simulink model "CAMFC2_01_WMR01"  (R2017b)
settings: Solver=ode45  StartTime=0.0  StopTime=150  RelTol=1e-3  EnableMultiTasking=on
InitFcn:
  | constant_CAMFC2_01_WMR01
values from neighbouring files (symbols this model uses):
  alpha = 0.1    [constant_CAMFC2_01_WMR01.m]    (also in constant_CAMFC2_04_Comp.m = 0.01; constant_CAMFC2_04_Quad_03.m; constant_CAMFC2_04_Simple.m = 0.01; constant_CAMFC2_04_Simple_DoubleIntegrator.m = 0.01)
  AN = [     0 1 0 0 ... (first row only)    [constant_CAMFC2_01_WMR01.m]    (also in constant_CAMFC2_04_Comp.m = [     0 1 0 0 1; constant_CAMFC2_04_Quad_03.m; constant_CAMFC2_04_Simple.m; constant_CAMFC2_04_Simple_DoubleIntegrator.m)
  B = eye(n)    [constant_CAMFC2_01_WMR01.m]    (also in constant_CAMFC2_04_Quad_03.m; constant_CAMFC2_Quad_New_02.m)
  B_pseudo_inverse = ((B'*B)^(-1))*B'    [constant_CAMFC2_01_WMR01.m]    (also in constant_CAMFC2_Quad_New_02.m)
  BN = [     1 0 0 0 ... (first row only)    [constant_CAMFC2_01_WMR01.m]    (also in constant_CAMFC2_04_Comp.m = [     0 0 0 0 0; constant_CAMFC2_04_Quad_03.m; constant_CAMFC2_04_Simple.m; constant_CAMFC2_04_Simple_DoubleIntegrator.m)
  chi = [0 0 0 0 ... (first row only)    [constant_CAMFC2_01_WMR01.m]    (also in constant_CAMFC2_04_Comp.m = X_m*ones(n0,1); constant_CAMFC2_04_Quad_03.m = X_m*ones(n0,1); constant_CAMFC2_04_Simple.m = X_m*ones(n0,1); constant_CAMFC2_04_Simple_DoubleIntegrator.m = X_m*ones(n0,1))
  Cv = 0.1    [constant_CAMFC2_01_WMR01.m]
  Cw = 0.1    [constant_CAMFC2_01_WMR01.m]
  epsilon_struct = struct('data',epsilon_InitVal)    [constant_CAMFC2_01_WMR01.m]    (also in constant_CAMFC2_04_Comp.m; constant_CAMFC2_04_Quad_03.m; constant_CAMFC2_04_Simple.m; constant_CAMFC2_04_Simple_DoubleIntegrator.m)
  gama1 = 1e4*diag([1e-6*ones(2,1);1e0*ones(2,1)])    [constant_CAMFC2_01_WMR01.m]    (also in constant_CAMFC2_04_Comp.m = 1e+3*diag([1e-6;1e-0]); constant_CAMFC2_04_Quad_03.m = 1e+2*diag(1e-0*ones(n0,1)); constant_CAMFC2_04_Simple.m = 1e+2*diag([1e-0;1e-0]); constant_CAMFC2_04_Simple_Formation.m = 1e+2*diag([1e-0;1e-0]))
  gama2 = 1e-2*diag([1e-6*ones(2,1);1e0*ones(2,1)])    [constant_CAMFC2_01_WMR01.m]    (also in constant_CAMFC2_04_Comp.m = 1e+0*diag([1e-6;1e-0]); constant_CAMFC2_04_Quad_03.m = 1e+0*diag(1e-0*ones(n0,1)); constant_CAMFC2_04_Simple.m = 1e+1*diag([1e-0;1e-0]); constant_CAMFC2_04_Simple_Formation.m = 1e+1*diag([1e-0;1e-0]))
  H = L + BN    [constant_CAMFC2_01_WMR01.m]    (also in constant_CAMFC2_04_Comp.m; constant_CAMFC2_04_Quad_03.m; constant_CAMFC2_04_Simple.m; constant_CAMFC2_04_Simple_DoubleIntegrator.m)
  J = 0.01    [constant_CAMFC2_01_WMR01.m]    (also in constant_CAMFC2_04_Quad_03.m = 1.0e-3 * diag([1 1 2],0); constant_CAMFC2_Quad_New_02.m = 1.2416e-3 * diag([1 1 2],0))
  K = 1e-2*eye(n)    [constant_CAMFC2_01_WMR01.m]    (also in constant_CAMFC2_Quad_New_02.m = 1e+1*eye(n))
  k1 = 1    [constant_CAMFC2_01_WMR01.m]    (also in constant_CAMFC2_04_Comp.m; constant_CAMFC2_04_Quad_03.m = 50; constant_CAMFC2_04_Simple.m; constant_CAMFC2_04_Simple_DoubleIntegrator.m)
  k2 = 1    [constant_CAMFC2_01_WMR01.m]    (also in constant_CAMFC2_04_Comp.m; constant_CAMFC2_04_Quad_03.m; constant_CAMFC2_04_Simple.m; constant_CAMFC2_04_Simple_DoubleIntegrator.m)
  L0 = 0.1    [constant_CAMFC2_01_WMR01.m]
  M = 1    [constant_CAMFC2_01_WMR01.m]    (also in constant_CAMFC2_04_Quad_03.m = 2; constant_CAMFC2_Quad_New_02.m = 2)
  N = 4    [constant_CAMFC2_01_WMR01.m]    (also in constant_CAMFC2_04_Comp.m = 5; constant_CAMFC2_04_Quad_03.m; constant_CAMFC2_04_Simple.m; constant_CAMFC2_04_Simple_DoubleIntegrator.m)
  n = 4    [constant_CAMFC2_01_WMR01.m]    (also in constant_CAMFC2_04_Comp.m = 2; constant_CAMFC2_04_Quad_03.m = 6; constant_CAMFC2_04_Simple.m = 2; constant_CAMFC2_04_Simple_DoubleIntegrator.m = 2)
  n0 = 2    [constant_CAMFC2_01_WMR01.m]    (also in constant_CAMFC2_04_Comp.m = 1; constant_CAMFC2_04_Quad_03.m = 3; constant_CAMFC2_04_Simple.m; constant_CAMFC2_04_Simple_DoubleIntegrator.m = 1)
  Observer_Gain = 100    [constant_CAMFC2_01_WMR01.m]    (also in constant_CAMFC2_04_Comp.m = 10; constant_CAMFC2_04_Quad_03.m = 1; constant_CAMFC2_04_Simple.m; constant_CAMFC2_04_Simple_DoubleIntegrator.m)
  Observer_Gain1 = 100    [constant_CAMFC2_01_WMR01.m]    (also in constant_CAMFC2_04_Comp.m = 10; constant_CAMFC2_04_Quad_03.m = 1; constant_CAMFC2_04_Simple.m; constant_CAMFC2_04_Simple_DoubleIntegrator.m)
  P_struct = struct('data',P_InitVal)    [constant_CAMFC2_01_WMR01.m]    (also in constant_CAMFC2_04_Comp.m; constant_CAMFC2_04_Quad_03.m; constant_CAMFC2_04_Simple.m; constant_CAMFC2_04_Simple_DoubleIntegrator.m)
  Q = 1e-0*eye(n)    [constant_CAMFC2_01_WMR01.m]    (also in constant_CAMFC2_04_Comp.m = 1.0e+2*eye(n); constant_CAMFC2_04_Quad_03.m = 1e-0*eye(n0); constant_CAMFC2_04_Simple.m = 1.0e+1*eye(n); constant_CAMFC2_04_Simple_Formation.m = 1.0e+1*eye(n))
  R = 1e-0*eye(n)    [constant_CAMFC2_01_WMR01.m]    (also in constant_CAMFC2_04_Quad_03.m; constant_CAMFC2_Quad_New_02.m = 1e+0*eye(n))
  R0 = 0.1    [constant_CAMFC2_01_WMR01.m]
  rho1 = 1e-1    (= 0.1)    [constant_CAMFC2_01_WMR01.m]    (also in constant_CAMFC2_04_Comp.m = 1; constant_CAMFC2_04_Quad_03.m = 1; constant_CAMFC2_04_Simple.m = 1; constant_CAMFC2_04_Simple_DoubleIntegrator.m = 1)
  rho2 = 1e-3    (= 0.001)    [constant_CAMFC2_01_WMR01.m]    (also in constant_CAMFC2_04_Comp.m = 1; constant_CAMFC2_04_Quad_03.m = 1; constant_CAMFC2_04_Simple.m = 1; constant_CAMFC2_04_Simple_DoubleIntegrator.m = 10)
  T_struct = struct('data',T_InitVal)    [constant_CAMFC2_01_WMR01.m]    (also in constant_CAMFC2_04_Comp.m; constant_CAMFC2_04_Quad_03.m; constant_CAMFC2_04_Simple.m; constant_CAMFC2_04_Simple_DoubleIntegrator.m)
  Thresh = 1e-4    (= 0.0001)    [constant_CAMFC2_01_WMR01.m]
  U_dot0_M = U_dot0_m*ones(n,1)    [constant_CAMFC2_01_WMR01.m]    (also in constant_CAMFC2_Quad_New_02.m = U_dot0_m*ones(n0,1))
  Upsilon_M = Upsilon_m*ones(n,1)    [constant_CAMFC2_01_WMR01.m]    (also in constant_CAMFC2_04_Comp.m; constant_CAMFC2_04_Quad_03.m = Upsilon_m*ones(n0,1); constant_CAMFC2_04_Simple.m; constant_CAMFC2_04_Simple_DoubleIntegrator.m)
libraries: simulink x1
(part 2 of 2)

== matlab function CAMFC2_01_WMR01/Agent #1/Decenteralized Cooperaive Controller #1/Differentiator2/Sliding differentiator ==
  data: u output; u1 input; e input; k1 parameter; alpha parameter
function u = fcn(u1,e,k1,alpha)

b=k1;

ABS = abs(e);
SGN = e ./ (ABS + alpha);
u = u1 - b*((ABS.^0.5).*SGN); 

end

== matlab function CAMFC2_01_WMR01/Agent #1/Decenteralized Cooperaive Controller #1/Differentiator2/Sliding differentiator1 ==
  data: Du1 output; e input; k2 parameter; alpha parameter
function Du1 = fcn(e,k2,alpha)

a=k2;

ABS = abs(e);
SGN = e ./ (ABS + alpha);
Du1 = - a*SGN;

end

== matlab function CAMFC2_01_WMR01/Agent #1/WMR Plant-01/WMR model ==
  data: X input; u1 input; DX output; u2 input; t input; Cv parameter; Cw parameter; M parameter; J parameter; R0 parameter; L0 parameter
function DX = fcn(X,u1,u2,t,Cv,Cw,M,J,R0,L0)

x = X(1);
y = X(2);
T = X(3);
v = X(4);
w = X(5);

T1 = 0.01 * u1; 
T2 = 0.01 * u2; 

F = (1/R0)*(T1+T2);
Tau = (L0/R0)*(T1-T2);

Dv = (F - Cv*v + (0*sin(1*t)))/M ;
Dw = (Tau - Cw*w + (0*sin(1*t)))/J ;

Dx = v*cos(T);
Dy = v*sin(T);
DT = w;

DX = [Dx Dy DT Dv Dw]';

end

== matlab function CAMFC2_01_WMR01/Agent #2/Controller interpreter ==
  data: u output; U input
function u = fcn(U)

U1 = U(3);
U2 = U(4); 

u1 = 0.5 * (U1+U2);
u2 = 0.5 * (U1-U2);

u = [u1;u2];

end

== matlab function CAMFC2_01_WMR01/Agent #1/Decenteralized Cooperaive Controller #1/Main Controller #1 ==
  data: n parameter; n0 parameter; U output; R parameter; Q parameter; P_i input; e_i input; K parameter; Zeta_i input; BN parameter; A_hat_i input; u0 input; z0 input; DT_i input; T_i input; N parameter; H parameter; B parameter; g_hat input; Approx_U input; Agent_Num input; B_pseudo_inverse parameter; ui input; x input
function U = fcn(n,n0,R,Q,P_i,e_i,K,Zeta_i,BN,A_hat_i,u0,z0,DT_i,T_i,N,H,B,g_hat,Approx_U,Agent_Num,B_pseudo_inverse,ui,x)

D_eta_0 = DT_i(1,:)';

%%
z0_i = [z0;ui(1:n0)];
u0_i = u0;

%%
U2 = 1/2 * R * P_i * e_i; %Consensus Error
U6 = - BN(Agent_Num,Agent_Num)*(D_eta_0 - u0_i); %Connection to the leader
U7 = K * Zeta_i; %Consensus time-integral

U1 = zeros(n,1);
U3 = BN(Agent_Num,Agent_Num)*z0_i - e_i;
U4 = zeros(n,1);
U5 = zeros(n,1);
for i=1:N      
    if i~= Agent_Num
        U1 = U1 - (H(Agent_Num,i)*B*Approx_U((i-1)*n+1:(i*n),1)); %Observer on leader
    end
    U3 = U3 + (H(Agent_Num,i)*(2*x((i-1)*n+1:(i*n),1)) - T_i(i+1,:)'); %Formation parameters  
    U4 = U4 - (H(Agent_Num,i)*g_hat((i-1)*n+1:(i*n),1)); %nonlinear compensation 
    U5 = U5 + (H(Agent_Num,i)*DT_i(i+1,:)'); %Derivative of Formation parameters  
end
U3 = -A_hat_i * U3;
U8 = (2*Q - 3/4*R*P_i)*e_i;

U_input = U1 + U2 + U3 + U4 + U5 + U6 + U7 + U8;

U = B_pseudo_inverse * U_input / H(Agent_Num,Agent_Num);

end

== matlab function CAMFC2_01_WMR01/Agent #1/Decenteralized Cooperaive Controller #1/Module to compute Consensus Error #1 ==
  data: T_i input; xi input; x input; x0 input; ep output; AN parameter; BN parameter; N parameter; n parameter; n0 parameter; Agent_Num input; ui input; u0 input; Thresh parameter; xmi output; xm0 output; Td_in input; Td output
function [ep,xmi,xm0,Td] = fcn(T_i,xi,x,x0,AN,BN,N,n,n0,Agent_Num,ui,u0,Thresh,Td_in)

Diff_Star_to0 = (T_i((Agent_Num+1),:))';
Diff_Star_to_Other = (eye(n) * Diff_Star_to0 * ones(1,N))' - T_i(2:N+1,:);
Diff_Star_to_Other = Diff_Star_to_Other';

xp = zeros(n+1,N);
for i=1:N
    xp(1:n+1,i) = x((i-1)*(n+1)+1:(i*(n+1)));
end

%% variables modification

Ta = xi(3);
Td0 = Td_in(1);
if (abs(u0(1))+abs(u0(2))) > (1*Thresh)
    y_Err = (x0(2)-xi(2));
    x_Err = (x0(1)-xi(1));
    XS = (y_Err/x_Err);
    Td0 = atan(XS); 
    if abs(Td0)>1.5
        Td0 = abs(Td0);
    end
end

%Td = zeros(N+1,1);
%Td(1) = Td0;
Td = Td0;
Diff_Real = zeros(n,N);
Dxi = zeros(2,N);
for i=1:N
    Diff_Real(1,i) = (xp(1,Agent_Num) - xp(1,i))*cos(Ta) + (xp(2,Agent_Num) - xp(2,i))*sin(Ta);
%    Tdi = Td_in(i+1);
%     Dxi(1,i) = xp(4,i)*cos(xp(3,i));
%     Dxi(2,i) = xp(4,i)*sin(xp(3,i));
%     if (abs(Dxi(1,i))+abs(Dxi(2,i))) > Thresh
%         y_Erri = xp(2,Agent_Num) - xp(2,i);
%         x_Erri = xp(1,Agent_Num) - xp(1,i);
%         Tdi = atan(y_Erri/x_Erri);
%         if abs(Tdi)>1.5
%             Tdi = abs(Tdi);
%         end
%     end
%    Diff_Real(2,i) = Ta - Tdi;
    Diff_Real(2,i) = Ta - xp(3,i);
    Diff_Real(3:4,i) = xp(4:5,Agent_Num) - xp(4:5,i); 
%    Td(i+1) = Tdi;
end
Diff_Real0 = zeros(n,1);
Diff_Real0(1) = (xp(1,Agent_Num) - x0(1))*cos(Ta) + (xp(2,Agent_Num) - x0(2))*sin(Ta);
Diff_Real0(2) = Ta - Td0; 
Diff_Real0(3:4) = xp(4:5,Agent_Num) - ui(1:n0);

Posi = xi(1)*cos(Ta) + xi(2)*sin(Ta);
Posd = x0(1)*cos(Ta) + x0(2)*sin(Ta);
xmi = [Posi;Ta;xi(4);xi(5)];
xm0 = [Posd;Td0]; 

%%

ep = zeros(n,1);
ep(1:2,1) = ep(1:2,1) + ( BN(Agent_Num,Agent_Num)*(-Diff_Real0(1:2)+Diff_Star_to0(1:2)) );
ep(3:4,1) = ep(3:4,1) + ( 1*(-Diff_Real0(3:4)+Diff_Star_to0(3:4)) );
for i=1:N            
    ep(1:n,1) = ep(1:n,1) + AN(Agent_Num,i)*(-Diff_Real(:,i)+Diff_Star_to_Other(:,i));
end

end

== matlab function CAMFC2_01_WMR01/Agent #1/Decenteralized Cooperaive Controller #1/Observer T#1 ==
  data: T_struct parameter; T input; DT_i output; epsilon input; epsilon_struct parameter; H parameter; BN parameter; AN parameter; T_i input; chi parameter; Upsilon_M parameter; epsilon_i output; N parameter; n parameter; Agent_Num input; Observer_Gain1 parameter
function [DT_i,epsilon_i] = fcn(T_struct,T,epsilon,epsilon_struct,H,BN,AN,T_i,chi,Upsilon_M,N,n,Agent_Num,Observer_Gain1)

T_struct(1).data = T.t1;
T_struct(2).data = T.t2;
T_struct(3).data = T.t3;
T_struct(4).data = T.t4;

epsilon_struct(1).data = epsilon.eps1;
epsilon_struct(2).data = epsilon.eps2;
epsilon_struct(3).data = epsilon.eps3;
epsilon_struct(4).data = epsilon.eps4;

epsilon_i = + BN(Agent_Num,Agent_Num)*(T_i - chi);
Sum2 = zeros(N+1,n);
for i=1:N
    epsilon_i = epsilon_i + ( AN(Agent_Num,i) * (T_i - T_struct(i).data) );  
    Sum2 = Sum2 + ( H(i,Agent_Num) * epsilon_struct(i).data );
end

Sum21 = abs(Sum2) + 0.1;
SGN2 = Sum2./Sum21;

DT_i = -Observer_Gain1*epsilon_i - SGN2*diag(Upsilon_M);

end

== matlab function CAMFC2_01_WMR01/Agent #1/Decenteralized Cooperaive Controller #1/Observer q#1 ==
  data: q input; Dq_i output; tau input; H parameter; BN parameter; AN parameter; q_i input; u0 input; U_dot0_M parameter; tau_i output; N parameter; Agent_Num input; Observer_Gain parameter; n parameter
function [Dq_i,tau_i] = fcn(q,tau,H,BN,AN,q_i,u0,U_dot0_M,N,Agent_Num,Observer_Gain,n)

tau_i = + BN(Agent_Num,Agent_Num)*(q_i - u0);
Sum2 = zeros(n,1);
for i=1:N
    tau_i = tau_i + ( AN(Agent_Num,i) * (q_i - q(((i-1)*n+1):n*i)) );  
    Sum2 = Sum2 + ( H(i,Agent_Num) * tau(((i-1)*n+1):n*i) );
end

Sum21 = abs(Sum2) + 0.01;
SGN2 = Sum2./Sum21;

Dq_i = -Observer_Gain*tau_i - diag(SGN2)*U_dot0_M;

end

== matlab function CAMFC2_01_WMR01/Agent #1/Decenteralized Cooperaive Controller #1/DRE ==
  data: P input; A_hat input; B parameter; R parameter; DP output; Q parameter
function DP = fcn(P,A_hat,B,R,Q)

DP = 2*A_hat*P + 2*P*A_hat' - P*B*R*B'*P + 2*Q;

end

== matlab function CAMFC2_01_WMR01/Agent #2/WMR Plant-02/WMR model ==
  data: X input; u1 input; DX output; u2 input; t input; Cv parameter; Cw parameter; M parameter; J parameter; R0 parameter; L0 parameter
function DX = fcn(X,u1,u2,t,Cv,Cw,M,J,R0,L0)

x = X(1);
y = X(2);
T = X(3);
v = X(4);
w = X(5);

T1 = 0.01 * u1; 
T2 = 0.01 * u2; 

F = (1/R0)*(T1+T2);
Tau = (L0/R0)*(T1-T2);

Dv = (F - Cv*v + (0*sin(1*t)))/M ;
Dw = (Tau - Cw*w + (0*sin(1*t)))/J ;

Dx = v*cos(T);
Dy = v*sin(T);
DT = w;

DX = [Dx Dy DT Dv Dw]';

end

== matlab function CAMFC2_01_WMR01/Agent #3/Controller interpreter ==
  data: u output; U input
function u = fcn(U)

U1 = U(3);
U2 = U(4); 

u1 = 0.5 * (U1+U2);
u2 = 0.5 * (U1-U2);

u = [u1;u2];

end

== matlab function CAMFC2_01_WMR01/Agent #2/Decenteralized Cooperaive Controller #2/Adaptive Law A#2 ==
  data: Agent_Num input; A_hat input; gama2 parameter; rho2 parameter; T_i input; P_i input; DA_hat output; e_i input; H parameter; BN parameter; N parameter; n parameter; n0 parameter; z0 input; x input; ui input
function DA_hat = fcn(Agent_Num,A_hat,gama2,rho2,T_i,P_i,e_i,H,BN,N,n,n0,z0,x,ui)

%% 
z0_i = [z0;ui(1:n0)]; 

%%
vA_hat = diag(A_hat);

Sum = zeros(n,1);
for i=2:(N+1)
    Sum = Sum + (H(Agent_Num,(i-1)) * (2*x(((i-1)-1)*n+1:((i-1)*n),1)) - T_i(i,:)');
end
Sum = Sum + BN(Agent_Num,Agent_Num)*z0_i - e_i;
    
DvA_hat = -gama2*diag(Sum)*P_i * e_i - (rho2*gama2*vA_hat);

DA_hat = diag(DvA_hat);

end

== matlab function CAMFC2_01_WMR01/Agent #2/Decenteralized Cooperaive Controller #2/Adaptive Law g#2 ==
  data: Agent_Num input; g_hat input; gama1 parameter; rho1 parameter; P input; P_struct parameter; Dg_hat output; e input; H parameter; N parameter; n parameter
function Dg_hat = fcn(Agent_Num,g_hat,gama1,rho1,P,P_struct,e,H,N,n)

P_struct(1).data = P.p1;
P_struct(2).data = P.p2;
P_struct(3).data = P.p3;
P_struct(4).data = P.p4;

Sum = zeros(n,1);
for i=1:N  
    Sum = Sum + (H(i,Agent_Num) * P_struct(i).data * e((i-1)*n+1:(i*n),1)); %Adaptive law
end
    
Dg_hat = -gama1*Sum - (rho1*gama1*g_hat);

end

== matlab function CAMFC2_01_WMR01/Agent #2/Decenteralized Cooperaive Controller #2/Approx. U#2 ==
  data: Agent_Num input; q_i input; DT_i input; Approx_U_i output; B_pseudo_inverse parameter; A_hat_i input; x_i input; g_hat_i input
function Approx_U_i  = fcn(Agent_Num,q_i,DT_i,B_pseudo_inverse,A_hat_i,x_i,g_hat_i)

D_eta_0 = DT_i(1,:)';
D_eta_i = DT_i(Agent_Num,:)';

u0_i = q_i;

Approx_U_i = B_pseudo_inverse * (u0_i - A_hat_i * x_i - g_hat_i + D_eta_i - D_eta_0);

end

== matlab function CAMFC2_01_WMR01/Agent #2/Decenteralized Cooperaive Controller #2/DRE ==
  data: P input; A_hat input; B parameter; R parameter; DP output; Q parameter
function DP = fcn(P,A_hat,B,R,Q)

DP = 2*A_hat*P + 2*P*A_hat' - P*B*R*B'*P + 2*Q;

end

== matlab function CAMFC2_01_WMR01/Agent #1/Decenteralized Cooperaive Controller #1/Differentiator1/Sliding differentiator ==
  data: u output; u1 input; e input; k1 parameter; alpha parameter
function u = fcn(u1,e,k1,alpha)

b=k1;

ABS = abs(e);
SGN = e ./ (ABS + alpha);
u = u1 - b*((ABS.^0.5).*SGN); 

end

== matlab function CAMFC2_01_WMR01/Agent #1/Decenteralized Cooperaive Controller #1/Differentiator1/Sliding differentiator1 ==
  data: Du1 output; e input; k2 parameter; alpha parameter
function Du1 = fcn(e,k2,alpha)

a=k2;

ABS = abs(e);
SGN = e ./ (ABS + alpha);
Du1 = - a*SGN;

end

== matlab function CAMFC2_01_WMR01/Agent #3/WMR Plant-03/WMR model ==
  data: X input; u1 input; DX output; u2 input; t input; Cv parameter; Cw parameter; M parameter; J parameter; R0 parameter; L0 parameter
function DX = fcn(X,u1,u2,t,Cv,Cw,M,J,R0,L0)

x = X(1);
y = X(2);
T = X(3);
v = X(4);
w = X(5);

T1 = 0.01 * u1; 
T2 = 0.01 * u2; 

F = (1/R0)*(T1+T2);
Tau = (L0/R0)*(T1-T2);

Dv = (F - Cv*v + (0*sin(1*t)))/M ;
Dw = (Tau - Cw*w + (0*sin(1*t)))/J ;

Dx = v*cos(T);
Dy = v*sin(T);
DT = w;

DX = [Dx Dy DT Dv Dw]';

end

== matlab function CAMFC2_01_WMR01/Agent #4/Controller interpreter ==
  data: u output; U input
function u = fcn(U)

U1 = U(3);
U2 = U(4); 

u1 = 0.5 * (U1+U2);
u2 = 0.5 * (U1-U2);

u = [u1;u2];

end

== matlab function CAMFC2_01_WMR01/Agent #2/Decenteralized Cooperaive Controller #2/Differentiator0/Sliding differentiator ==
  data: u output; u1 input; e input; k1 parameter; alpha parameter
function u = fcn(u1,e,k1,alpha)

b=k1;

ABS = abs(e);
SGN = e ./ (ABS + alpha);
u = u1 - b*((ABS.^0.5).*SGN); 

end

== matlab function CAMFC2_01_WMR01/Agent #2/Decenteralized Cooperaive Controller #2/Differentiator0/Sliding differentiator1 ==
  data: Du1 output; e input; k2 parameter; alpha parameter
function Du1 = fcn(e,k2,alpha)

a=k2;

ABS = abs(e);
SGN = e ./ (ABS + alpha);
Du1 = - a*SGN;

end

== matlab function CAMFC2_01_WMR01/Agent #2/Decenteralized Cooperaive Controller #2/Differentiator1/Sliding differentiator ==
  data: u output; u1 input; e input; k1 parameter; alpha parameter
function u = fcn(u1,e,k1,alpha)

b=k1;

ABS = abs(e);
SGN = e ./ (ABS + alpha);
u = u1 - b*((ABS.^0.5).*SGN); 

end

== matlab function CAMFC2_01_WMR01/Agent #2/Decenteralized Cooperaive Controller #2/Differentiator1/Sliding differentiator1 ==
  data: Du1 output; e input; k2 parameter; alpha parameter
function Du1 = fcn(e,k2,alpha)

a=k2;

ABS = abs(e);
SGN = e ./ (ABS + alpha);
Du1 = - a*SGN;

end

== matlab function CAMFC2_01_WMR01/Agent #4/WMR Plant-04/WMR model ==
  data: X input; u1 input; DX output; u2 input; t input; Cv parameter; Cw parameter; M parameter; J parameter; R0 parameter; L0 parameter
function DX = fcn(X,u1,u2,t,Cv,Cw,M,J,R0,L0)

x = X(1);
y = X(2);
T = X(3);
v = X(4);
w = X(5);

T1 = 0.01 * u1; 
T2 = 0.01 * u2; 

F = (1/R0)*(T1+T2);
Tau = (L0/R0)*(T1-T2);

Dv = (F - Cv*v + (0*sin(1*t)))/M ;
Dw = (Tau - Cw*w + (0*sin(1*t)))/J ;

Dx = v*cos(T);
Dy = v*sin(T);
DT = w;

DX = [Dx Dy DT Dv Dw]';

end

== matlab function CAMFC2_01_WMR01/Agent #2/Decenteralized Cooperaive Controller #2/Differentiator2/Sliding differentiator ==
  data: u output; u1 input; e input; k1 parameter; alpha parameter
function u = fcn(u1,e,k1,alpha)

b=k1;

ABS = abs(e);
SGN = e ./ (ABS + alpha);
u = u1 - b*((ABS.^0.5).*SGN); 

end

== matlab function CAMFC2_01_WMR01/Agent #3/Decenteralized Cooperaive Controller #3/Adaptive Law A#3 ==
  data: Agent_Num input; A_hat input; gama2 parameter; rho2 parameter; T_i input; P_i input; DA_hat output; e_i input; H parameter; BN parameter; N parameter; n parameter; n0 parameter; z0 input; x input; ui input
function DA_hat = fcn(Agent_Num,A_hat,gama2,rho2,T_i,P_i,e_i,H,BN,N,n,n0,z0,x,ui)

%% 
z0_i = [z0;ui(1:n0)]; 

%%
vA_hat = diag(A_hat);

Sum = zeros(n,1);
for i=2:(N+1)
    Sum = Sum + (H(Agent_Num,(i-1)) * (2*x(((i-1)-1)*n+1:((i-1)*n),1)) - T_i(i,:)');
end
Sum = Sum + BN(Agent_Num,Agent_Num)*z0_i - e_i;
    
DvA_hat = -gama2*diag(Sum)*P_i * e_i - (rho2*gama2*vA_hat);

DA_hat = diag(DvA_hat);

end

== matlab function CAMFC2_01_WMR01/Agent #3/Decenteralized Cooperaive Controller #3/Adaptive Law g#3 ==
  data: Agent_Num input; g_hat input; gama1 parameter; rho1 parameter; P input; P_struct parameter; Dg_hat output; e input; H parameter; N parameter; n parameter
function Dg_hat = fcn(Agent_Num,g_hat,gama1,rho1,P,P_struct,e,H,N,n)

P_struct(1).data = P.p1;
P_struct(2).data = P.p2;
P_struct(3).data = P.p3;
P_struct(4).data = P.p4;

Sum = zeros(n,1);
for i=1:N  
    Sum = Sum + (H(i,Agent_Num) * P_struct(i).data * e((i-1)*n+1:(i*n),1)); %Adaptive law
end
    
Dg_hat = -gama1*Sum - (rho1*gama1*g_hat);

end

== matlab function CAMFC2_01_WMR01/Agent #3/Decenteralized Cooperaive Controller #3/Approx. U#3 ==
  data: Agent_Num input; q_i input; DT_i input; Approx_U_i output; B_pseudo_inverse parameter; A_hat_i input; x_i input; g_hat_i input
function Approx_U_i  = fcn(Agent_Num,q_i,DT_i,B_pseudo_inverse,A_hat_i,x_i,g_hat_i)

D_eta_0 = DT_i(1,:)';
D_eta_i = DT_i(Agent_Num,:)';

u0_i = q_i;

Approx_U_i = B_pseudo_inverse * (u0_i - A_hat_i * x_i - g_hat_i + D_eta_i - D_eta_0);

end

== matlab function CAMFC2_01_WMR01/Agent #3/Decenteralized Cooperaive Controller #3/DRE ==
  data: P input; A_hat input; B parameter; R parameter; DP output; Q parameter
function DP = fcn(P,A_hat,B,R,Q)

DP = 2*A_hat*P + 2*P*A_hat' - P*B*R*B'*P + 2*Q;

end

== matlab function CAMFC2_01_WMR01/Agent #2/Decenteralized Cooperaive Controller #2/Differentiator2/Sliding differentiator1 ==
  data: Du1 output; e input; k2 parameter; alpha parameter
function Du1 = fcn(e,k2,alpha)

a=k2;

ABS = abs(e);
SGN = e ./ (ABS + alpha);
Du1 = - a*SGN;

end

== matlab function CAMFC2_01_WMR01/Agent #2/Decenteralized Cooperaive Controller #2/Main Controller #2 ==
  data: n parameter; n0 parameter; U output; R parameter; Q parameter; P_i input; e_i input; K parameter; Zeta_i input; BN parameter; A_hat_i input; u0 input; z0 input; DT_i input; T_i input; N parameter; H parameter; B parameter; g_hat input; Approx_U input; Agent_Num input; B_pseudo_inverse parameter; ui input; x input
function U = fcn(n,n0,R,Q,P_i,e_i,K,Zeta_i,BN,A_hat_i,u0,z0,DT_i,T_i,N,H,B,g_hat,Approx_U,Agent_Num,B_pseudo_inverse,ui,x)

D_eta_0 = DT_i(1,:)';

%%
z0_i = [z0;ui(1:n0)];
u0_i = u0;

%%
U2 = 1/2 * R * P_i * e_i; %Consensus Error
U6 = - BN(Agent_Num,Agent_Num)*(D_eta_0 - u0_i); %Connection to the leader
U7 = K * Zeta_i; %Consensus time-integral

U1 = zeros(n,1);
U3 = BN(Agent_Num,Agent_Num)*z0_i - e_i;
U4 = zeros(n,1);
U5 = zeros(n,1);
for i=1:N      
    if i~= Agent_Num
        U1 = U1 - (H(Agent_Num,i)*B*Approx_U((i-1)*n+1:(i*n),1)); %Observer on leader
    end
    U3 = U3 + (H(Agent_Num,i)*(2*x((i-1)*n+1:(i*n),1)) - T_i(i+1,:)'); %Formation parameters  
    U4 = U4 - (H(Agent_Num,i)*g_hat((i-1)*n+1:(i*n),1)); %nonlinear compensation 
    U5 = U5 + (H(Agent_Num,i)*DT_i(i+1,:)'); %Derivative of Formation parameters  
end
U3 = -A_hat_i * U3;
U8 = (2*Q - 3/4*R*P_i)*e_i;

U_input = U1 + U2 + U3 + U4 + U5 + U6 + U7 + U8;

U = B_pseudo_inverse * U_input / H(Agent_Num,Agent_Num);

end

== matlab function CAMFC2_01_WMR01/Agent #1/Decenteralized Cooperaive Controller #1/Differentiator0/Sliding differentiator ==
  data: u output; u1 input; e input; k1 parameter; alpha parameter
function u = fcn(u1,e,k1,alpha)

b=k1;

ABS = abs(e);
SGN = e ./ (ABS + alpha);
u = u1 - b*((ABS.^0.5).*SGN); 

end

== matlab function CAMFC2_01_WMR01/Agent #1/Decenteralized Cooperaive Controller #1/Differentiator0/Sliding differentiator1 ==
  data: Du1 output; e input; k2 parameter; alpha parameter
function Du1 = fcn(e,k2,alpha)

a=k2;

ABS = abs(e);
SGN = e ./ (ABS + alpha);
Du1 = - a*SGN;

end

== matlab function CAMFC2_01_WMR01/Agent #3/Decenteralized Cooperaive Controller #3/Differentiator0/Sliding differentiator ==
  data: u output; u1 input; e input; k1 parameter; alpha parameter
function u = fcn(u1,e,k1,alpha)

b=k1;

ABS = abs(e);
SGN = e ./ (ABS + alpha);
u = u1 - b*((ABS.^0.5).*SGN); 

end

== matlab function CAMFC2_01_WMR01/Agent #3/Decenteralized Cooperaive Controller #3/Differentiator0/Sliding differentiator1 ==
  data: Du1 output; e input; k2 parameter; alpha parameter
function Du1 = fcn(e,k2,alpha)

a=k2;

ABS = abs(e);
SGN = e ./ (ABS + alpha);
Du1 = - a*SGN;

end

== matlab function CAMFC2_01_WMR01/Agent #3/Decenteralized Cooperaive Controller #3/Differentiator1/Sliding differentiator ==
  data: u output; u1 input; e input; k1 parameter; alpha parameter
function u = fcn(u1,e,k1,alpha)

b=k1;

ABS = abs(e);
SGN = e ./ (ABS + alpha);
u = u1 - b*((ABS.^0.5).*SGN); 

end

== matlab function CAMFC2_01_WMR01/Agent #3/Decenteralized Cooperaive Controller #3/Differentiator1/Sliding differentiator1 ==
  data: Du1 output; e input; k2 parameter; alpha parameter
function Du1 = fcn(e,k2,alpha)

a=k2;

ABS = abs(e);
SGN = e ./ (ABS + alpha);
Du1 = - a*SGN;

end

== matlab function CAMFC2_01_WMR01/Agent #3/Decenteralized Cooperaive Controller #3/Differentiator2/Sliding differentiator ==
  data: u output; u1 input; e input; k1 parameter; alpha parameter
function u = fcn(u1,e,k1,alpha)

b=k1;

ABS = abs(e);
SGN = e ./ (ABS + alpha);
u = u1 - b*((ABS.^0.5).*SGN); 

end

== matlab function CAMFC2_01_WMR01/Agent #3/Decenteralized Cooperaive Controller #3/Differentiator2/Sliding differentiator1 ==
  data: Du1 output; e input; k2 parameter; alpha parameter
function Du1 = fcn(e,k2,alpha)

a=k2;

ABS = abs(e);
SGN = e ./ (ABS + alpha);
Du1 = - a*SGN;

end

== matlab function CAMFC2_01_WMR01/Agent #4/Decenteralized Cooperaive Controller #4/Adaptive Law A#4 ==
  data: Agent_Num input; A_hat input; gama2 parameter; rho2 parameter; T_i input; P_i input; DA_hat output; e_i input; H parameter; BN parameter; N parameter; n parameter; n0 parameter; z0 input; x input; ui input
function DA_hat = fcn(Agent_Num,A_hat,gama2,rho2,T_i,P_i,e_i,H,BN,N,n,n0,z0,x,ui)

%% 
z0_i = [z0;ui(1:n0)]; 

%%
vA_hat = diag(A_hat);

Sum = zeros(n,1);
for i=2:(N+1)
    Sum = Sum + (H(Agent_Num,(i-1)) * (2*x(((i-1)-1)*n+1:((i-1)*n),1)) - T_i(i,:)');
end
Sum = Sum + BN(Agent_Num,Agent_Num)*z0_i - e_i;
    
DvA_hat = -gama2*diag(Sum)*P_i * e_i - (rho2*gama2*vA_hat);

DA_hat = diag(DvA_hat);

end

== matlab function CAMFC2_01_WMR01/Agent #4/Decenteralized Cooperaive Controller #4/Adaptive Law g#4 ==
  data: Agent_Num input; g_hat input; gama1 parameter; rho1 parameter; P input; P_struct parameter; Dg_hat output; e input; H parameter; N parameter; n parameter
function Dg_hat = fcn(Agent_Num,g_hat,gama1,rho1,P,P_struct,e,H,N,n)

P_struct(1).data = P.p1;
P_struct(2).data = P.p2;
P_struct(3).data = P.p3;
P_struct(4).data = P.p4;

Sum = zeros(n,1);
for i=1:N  
    Sum = Sum + (H(i,Agent_Num) * P_struct(i).data * e((i-1)*n+1:(i*n),1)); %Adaptive law
end
    
Dg_hat = -gama1*Sum - (rho1*gama1*g_hat);

end

== matlab function CAMFC2_01_WMR01/Agent #4/Decenteralized Cooperaive Controller #4/Approx. U#4 ==
  data: Agent_Num input; q_i input; DT_i input; Approx_U_i output; B_pseudo_inverse parameter; A_hat_i input; x_i input; g_hat_i input
function Approx_U_i  = fcn(Agent_Num,q_i,DT_i,B_pseudo_inverse,A_hat_i,x_i,g_hat_i)

D_eta_0 = DT_i(1,:)';
D_eta_i = DT_i(Agent_Num,:)';

u0_i = q_i;

Approx_U_i = B_pseudo_inverse * (u0_i - A_hat_i * x_i - g_hat_i + D_eta_i - D_eta_0);

end

== matlab function CAMFC2_01_WMR01/Agent #4/Decenteralized Cooperaive Controller #4/DRE ==
  data: P input; A_hat input; B parameter; R parameter; DP output; Q parameter
function DP = fcn(P,A_hat,B,R,Q)

DP = 2*A_hat*P + 2*P*A_hat' - P*B*R*B'*P + 2*Q;

end

== matlab function CAMFC2_01_WMR01/Agent #4/Decenteralized Cooperaive Controller #4/Differentiator0/Sliding differentiator ==
  data: u output; u1 input; e input; k1 parameter; alpha parameter
function u = fcn(u1,e,k1,alpha)

b=k1;

ABS = abs(e);
SGN = e ./ (ABS + alpha);
u = u1 - b*((ABS.^0.5).*SGN); 

end

== matlab function CAMFC2_01_WMR01/Agent #4/Decenteralized Cooperaive Controller #4/Differentiator0/Sliding differentiator1 ==
  data: Du1 output; e input; k2 parameter; alpha parameter
function Du1 = fcn(e,k2,alpha)

a=k2;

ABS = abs(e);
SGN = e ./ (ABS + alpha);
Du1 = - a*SGN;

end

== matlab function CAMFC2_01_WMR01/Agent #2/Decenteralized Cooperaive Controller #2/Module to compute Consensus Error #2 ==
  data: T_i input; xi input; x input; x0 input; ep output; AN parameter; BN parameter; N parameter; n parameter; n0 parameter; Agent_Num input; ui input; u0 input; Thresh parameter; xmi output; xm0 output; Td_in input; Td output
function [ep,xmi,xm0,Td] = fcn(T_i,xi,x,x0,AN,BN,N,n,n0,Agent_Num,ui,u0,Thresh,Td_in)

Diff_Star_to0 = (T_i((Agent_Num+1),:))';
Diff_Star_to_Other = (eye(n) * Diff_Star_to0 * ones(1,N))' - T_i(2:N+1,:);
Diff_Star_to_Other = Diff_Star_to_Other';

xp = zeros(n+1,N);
for i=1:N
    xp(1:n+1,i) = x((i-1)*(n+1)+1:(i*(n+1)));
end

%% variables modification

Ta = xi(3);
Td0 = Td_in(1);
if (abs(u0(1))+abs(u0(2))) > (1*Thresh)
    y_Err = (x0(2)-xi(2));
    x_Err = (x0(1)-xi(1));
    XS = (y_Err/x_Err);
    Td0 = atan(XS); 
    if abs(Td0)>1.5
        Td0 = abs(Td0);
    end
end

% Td = zeros(N+1,1);
% Td(1) = Td0;
Td = Td0;
Diff_Real = zeros(n,N);
Dxi = zeros(2,N);
for i=1:N
    Diff_Real(1,i) = (xp(1,Agent_Num) - xp(1,i))*cos(Ta) + (xp(2,Agent_Num) - xp(2,i))*sin(Ta);
%     Tdi = Td_in(i+1);
%     Dxi(1,i) = xp(4,i)*cos(xp(3,i));
%     Dxi(2,i) = xp(4,i)*sin(xp(3,i));
%     if (abs(Dxi(1,i))+abs(Dxi(2,i))) > Thresh
%         y_Erri = xp(2,Agent_Num) - xp(2,i);
%         x_Erri = xp(1,Agent_Num) - xp(1,i);
%         Tdi = atan(y_Erri/x_Erri);
%         if abs(Tdi)>1.5
%             Tdi = abs(Tdi);
%         end
%     end
%     Diff_Real(2,i) = Ta - Tdi;
    Diff_Real(2,i) = Ta - xp(3,i);
    Diff_Real(3:4,i) = xp(4:5,Agent_Num) - xp(4:5,i); 
%    Td(i+1) = Tdi;
end
Diff_Real0 = zeros(n,1);
Diff_Real0(1) = (xp(1,Agent_Num) - x0(1))*cos(Ta) + (xp(2,Agent_Num) - x0(2))*sin(Ta);
Diff_Real0(2) = Ta - Td0; 
Diff_Real0(3:4) = xp(4:5,Agent_Num) - ui(1:n0);

Posi = xi(1)*cos(Ta) + xi(2)*sin(Ta);
Posd = x0(1)*cos(Ta) + x0(2)*sin(Ta);
xmi = [Posi;Ta;xi(4);xi(5)];
xm0 = [Posd;Td0]; 

%%

ep = zeros(n,1);
ep(1:2,1) = ep(1:2,1) + ( BN(Agent_Num,Agent_Num)*(-Diff_Real0(1:2)+Diff_Star_to0(1:2)) );
ep(3:4,1) = ep(3:4,1) + ( 1*(-Diff_Real0(3:4)+Diff_Star_to0(3:4)) );
for i=1:N            
    ep(1:n,1) = ep(1:n,1) + AN(Agent_Num,i)*(-Diff_Real(:,i)+Diff_Star_to_Other(:,i));
end

end

== matlab function CAMFC2_01_WMR01/Agent #2/Decenteralized Cooperaive Controller #2/Observer T#2 ==
  data: T_struct parameter; T input; DT_i output; epsilon input; epsilon_struct parameter; H parameter; BN parameter; AN parameter; T_i input; chi parameter; Upsilon_M parameter; epsilon_i output; N parameter; n parameter; Agent_Num input; Observer_Gain1 parameter
function [DT_i,epsilon_i] = fcn(T_struct,T,epsilon,epsilon_struct,H,BN,AN,T_i,chi,Upsilon_M,N,n,Agent_Num,Observer_Gain1)

T_struct(1).data = T.t1;
T_struct(2).data = T.t2;
T_struct(3).data = T.t3;
T_struct(4).data = T.t4;

epsilon_struct(1).data = epsilon.eps1;
epsilon_struct(2).data = epsilon.eps2;
epsilon_struct(3).data = epsilon.eps3;
epsilon_struct(4).data = epsilon.eps4;

epsilon_i = + BN(Agent_Num,Agent_Num)*(T_i - chi);
Sum2 = zeros(N+1,n);
for i=1:N
    epsilon_i = epsilon_i + ( AN(Agent_Num,i) * (T_i - T_struct(i).data) );  
    Sum2 = Sum2 + ( H(i,Agent_Num) * epsilon_struct(i).data );
end

Sum21 = abs(Sum2) + 0.1;
SGN2 = Sum2./Sum21;

DT_i = -Observer_Gain1*epsilon_i - SGN2*diag(Upsilon_M);

end

== matlab function CAMFC2_01_WMR01/Data Bus /Reference Trajectory/Desired States/MATLAB Function ==
  data: t input; y output
function y = fcn(t)

y = sin(0.2*t) + cos(0.5*t);

end

== matlab function CAMFC2_01_WMR01/Data Bus /Reference Trajectory/Differentiator0/Sliding differentiator ==
  data: u output; u1 input; e input; k1 parameter; alpha parameter
function u = fcn(u1,e,k1,alpha)

b=k1;

ABS = abs(e);
SGN = e ./ (ABS + alpha);
u = u1 - b*((ABS.^0.5).*SGN); 

end

== matlab function CAMFC2_01_WMR01/Data Bus /For matrix Plot1/MATLAB Function ==
  data: u input; y output
function y = fcn(u)
S1 = size(u,1);
S2 = size(u,2);

y = zeros(S1*S2,1);
num = 0;
for i=1:S1
    for j=1:S2
        num = num + 1;
        y(num,1) = u(i,j);
    end
end

end

== matlab function CAMFC2_01_WMR01/Data Bus /For matrix Plot2/MATLAB Function ==
  data: u input; y output
function y = fcn(u)
S1 = size(u,1);
S2 = size(u,2);

y = zeros(S1*S2,1);
num = 0;
for i=1:S1
    for j=1:S2
        num = num + 1;
        y(num,1) = u(i,j);
    end
end

end

== matlab function CAMFC2_01_WMR01/Data Bus /For matrix Plot3/MATLAB Function ==
  data: u input; y output
function y = fcn(u)
S1 = size(u,1);
S2 = size(u,2);

y = zeros(S1*S2,1);
num = 0;
for i=1:S1
    for j=1:S2
        num = num + 1;
        y(num,1) = u(i,j);
    end
end

end

== matlab function CAMFC2_01_WMR01/Data Bus /For matrix Plot4/MATLAB Function ==
  data: u input; y output
function y = fcn(u)
S1 = size(u,1);
S2 = size(u,2);

y = zeros(S1*S2,1);
num = 0;
for i=1:S1
    for j=1:S2
        num = num + 1;
        y(num,1) = u(i,j);
    end
end

end

== matlab function CAMFC2_01_WMR01/Data Bus /For matrix Plot5/MATLAB Function ==
  data: u input; y output
function y = fcn(u)
S1 = size(u,1);
S2 = size(u,2);

y = zeros(S1*S2,1);
num = 0;
for i=1:S1
    for j=1:S2
        num = num + 1;
        y(num,1) = u(i,j);
    end
end

end

== matlab function CAMFC2_01_WMR01/Data Bus /For matrix Plot6/MATLAB Function ==
  data: u input; y output
function y = fcn(u)
S1 = size(u,1);
S2 = size(u,2);

y = zeros(S1*S2,1);
num = 0;
for i=1:S1
    for j=1:S2
        num = num + 1;
        y(num,1) = u(i,j);
    end
end

end

== matlab function CAMFC2_01_WMR01/Data Bus /For matrix Plot7/MATLAB Function ==
  data: u input; y output
function y = fcn(u)
S1 = size(u,1);
S2 = size(u,2);

y = zeros(S1*S2,1);
num = 0;
for i=1:S1
    for j=1:S2
        num = num + 1;
        y(num,1) = u(i,j);
    end
end

end

== matlab function CAMFC2_01_WMR01/Data Bus /For matrix Plot8/MATLAB Function ==
  data: u input; y output
function y = fcn(u)
S1 = size(u,1);
S2 = size(u,2);

y = zeros(S1*S2,1);
num = 0;
for i=1:S1
    for j=1:S2
        num = num + 1;
        y(num,1) = u(i,j);
    end
end

end

== matlab function CAMFC2_01_WMR01/Data Bus /For matrix Plot9/MATLAB Function ==
  data: u input; y output
function y = fcn(u)
S1 = size(u,1);
S2 = size(u,2);

y = zeros(S1*S2,1);
num = 0;
for i=1:S1
    for j=1:S2
        num = num + 1;
        y(num,1) = u(i,j);
    end
end

end

== matlab function CAMFC2_01_WMR01/Agent #4/Decenteralized Cooperaive Controller #4/Differentiator1/Sliding differentiator ==
  data: u output; u1 input; e input; k1 parameter; alpha parameter
function u = fcn(u1,e,k1,alpha)

b=k1;

ABS = abs(e);
SGN = e ./ (ABS + alpha);
u = u1 - b*((ABS.^0.5).*SGN); 

end

== matlab function CAMFC2_01_WMR01/Agent #4/Decenteralized Cooperaive Controller #4/Differentiator1/Sliding differentiator1 ==
  data: Du1 output; e input; k2 parameter; alpha parameter
function Du1 = fcn(e,k2,alpha)

a=k2;

ABS = abs(e);
SGN = e ./ (ABS + alpha);
Du1 = - a*SGN;

end

== matlab function CAMFC2_01_WMR01/Data Bus /For matrix Plot/MATLAB Function ==
  data: u input; y output
function y = fcn(u)
S1 = size(u,1);
S2 = size(u,2);

y = zeros(S1*S2,1);
num = 0;
for i=1:S1
    for j=1:S2
        num = num + 1;
        y(num,1) = u(i,j);
    end
end

end

== matlab function CAMFC2_01_WMR01/Data Bus /For matrix Plot10/MATLAB Function ==
  data: u input; y output
function y = fcn(u)
S1 = size(u,1);
S2 = size(u,2);

y = zeros(S1*S2,1);
num = 0;
for i=1:S1
    for j=1:S2
        num = num + 1;
        y(num,1) = u(i,j);
    end
end

end

== matlab function CAMFC2_01_WMR01/Data Bus /For matrix Plot11/MATLAB Function ==
  data: u input; y output
function y = fcn(u)
S1 = size(u,1);
S2 = size(u,2);

y = zeros(S1*S2,1);
num = 0;
for i=1:S1
    for j=1:S2
        num = num + 1;
        y(num,1) = u(i,j);
    end
end

end

== matlab function CAMFC2_01_WMR01/Data Bus /For matrix Plot12/MATLAB Function ==
  data: u input; y output
function y = fcn(u)
S1 = size(u,1);
S2 = size(u,2);

y = zeros(S1*S2,1);
num = 0;
for i=1:S1
    for j=1:S2
        num = num + 1;
        y(num,1) = u(i,j);
    end
end

end

== matlab function CAMFC2_01_WMR01/Agent #4/Decenteralized Cooperaive Controller #4/Differentiator2/Sliding differentiator ==
  data: u output; u1 input; e input; k1 parameter; alpha parameter
function u = fcn(u1,e,k1,alpha)

b=k1;

ABS = abs(e);
SGN = e ./ (ABS + alpha);
u = u1 - b*((ABS.^0.5).*SGN); 

end

== matlab function CAMFC2_01_WMR01/Data Bus /For matrix Plot13/MATLAB Function ==
  data: u input; y output
function y = fcn(u)
S1 = size(u,1);
S2 = size(u,2);

y = zeros(S1*S2,1);
num = 0;
for i=1:S1
    for j=1:S2
        num = num + 1;
        y(num,1) = u(i,j);
    end
end

end

== matlab function CAMFC2_01_WMR01/Agent #4/Decenteralized Cooperaive Controller #4/Differentiator2/Sliding differentiator1 ==
  data: Du1 output; e input; k2 parameter; alpha parameter
function Du1 = fcn(e,k2,alpha)

a=k2;

ABS = abs(e);
SGN = e ./ (ABS + alpha);
Du1 = - a*SGN;

end

== matlab function CAMFC2_01_WMR01/Agent #2/Decenteralized Cooperaive Controller #2/Observer q#2 ==
  data: q input; Dq_i output; tau input; H parameter; BN parameter; AN parameter; q_i input; u0 input; U_dot0_M parameter; tau_i output; N parameter; Agent_Num input; Observer_Gain parameter; n parameter
function [Dq_i,tau_i] = fcn(q,tau,H,BN,AN,q_i,u0,U_dot0_M,N,Agent_Num,Observer_Gain,n)

tau_i = + BN(Agent_Num,Agent_Num)*(q_i - u0);
Sum2 = zeros(n,1);
for i=1:N
    tau_i = tau_i + ( AN(Agent_Num,i) * (q_i - q(((i-1)*n+1):n*i)) );  
    Sum2 = Sum2 + ( H(i,Agent_Num) * tau(((i-1)*n+1):n*i) );
end

Sum21 = abs(Sum2) + 0.01;
SGN2 = Sum2./Sum21;

Dq_i = -Observer_Gain*tau_i - diag(SGN2)*U_dot0_M;

end

== matlab function CAMFC2_01_WMR01/Data Bus /For matrix Plot14/MATLAB Function ==
  data: u input; y output
function y = fcn(u)
S1 = size(u,1);
S2 = size(u,2);

y = zeros(S1*S2,1);
num = 0;
for i=1:S1
    for j=1:S2
        num = num + 1;
        y(num,1) = u(i,j);
    end
end

end

== matlab function CAMFC2_01_WMR01/Data Bus /For matrix Plot15/MATLAB Function ==
  data: u input; y output
function y = fcn(u)
S1 = size(u,1);
S2 = size(u,2);

y = zeros(S1*S2,1);
num = 0;
for i=1:S1
    for j=1:S2
        num = num + 1;
        y(num,1) = u(i,j);
    end
end

end

== matlab function CAMFC2_01_WMR01/Data Bus /Reference Trajectory/Differentiator0/Sliding differentiator1 ==
  data: Du1 output; e input; k2 parameter; alpha parameter
function Du1 = fcn(e,k2,alpha)

a=k2;

ABS = abs(e);
SGN = e ./ (ABS + alpha);
Du1 = - a*SGN;

end

== matlab function CAMFC2_01_WMR01/Agent #3/Decenteralized Cooperaive Controller #3/Main Controller #3 ==
  data: n parameter; n0 parameter; U output; R parameter; Q parameter; P_i input; e_i input; K parameter; Zeta_i input; BN parameter; A_hat_i input; u0 input; z0 input; DT_i input; T_i input; N parameter; H parameter; B parameter; g_hat input; Approx_U input; Agent_Num input; B_pseudo_inverse parameter; ui input; x input
function U = fcn(n,n0,R,Q,P_i,e_i,K,Zeta_i,BN,A_hat_i,u0,z0,DT_i,T_i,N,H,B,g_hat,Approx_U,Agent_Num,B_pseudo_inverse,ui,x)

D_eta_0 = DT_i(1,:)';

%%
z0_i = [z0;ui(1:n0)];
u0_i = u0;

%%
U2 = 1/2 * R * P_i * e_i; %Consensus Error
U6 = - BN(Agent_Num,Agent_Num)*(D_eta_0 - u0_i); %Connection to the leader
U7 = K * Zeta_i; %Consensus time-integral

U1 = zeros(n,1);
U3 = BN(Agent_Num,Agent_Num)*z0_i - e_i;
U4 = zeros(n,1);
U5 = zeros(n,1);
for i=1:N      
    if i~= Agent_Num
        U1 = U1 - (H(Agent_Num,i)*B*Approx_U((i-1)*n+1:(i*n),1)); %Observer on leader
    end
    U3 = U3 + (H(Agent_Num,i)*(2*x((i-1)*n+1:(i*n),1)) - T_i(i+1,:)'); %Formation parameters  
    U4 = U4 - (H(Agent_Num,i)*g_hat((i-1)*n+1:(i*n),1)); %nonlinear compensation 
    U5 = U5 + (H(Agent_Num,i)*DT_i(i+1,:)'); %Derivative of Formation parameters  
end
U3 = -A_hat_i * U3;
U8 = (2*Q - 3/4*R*P_i)*e_i;

U_input = U1 + U2 + U3 + U4 + U5 + U6 + U7 + U8;

U = B_pseudo_inverse * U_input / H(Agent_Num,Agent_Num);

end

== matlab function CAMFC2_01_WMR01/Agent #3/Decenteralized Cooperaive Controller #3/Module to compute Consensus Error #3 ==
  data: T_i input; xi input; x input; x0 input; ep output; AN parameter; BN parameter; N parameter; n parameter; n0 parameter; Agent_Num input; ui input; u0 input; Thresh parameter; xmi output; xm0 output; Td_in input; Td output
function [ep,xmi,xm0,Td] = fcn(T_i,xi,x,x0,AN,BN,N,n,n0,Agent_Num,ui,u0,Thresh,Td_in)

Diff_Star_to0 = (T_i((Agent_Num+1),:))';
Diff_Star_to_Other = (eye(n) * Diff_Star_to0 * ones(1,N))' - T_i(2:N+1,:);
Diff_Star_to_Other = Diff_Star_to_Other';

xp = zeros(n+1,N);
for i=1:N
    xp(1:n+1,i) = x((i-1)*(n+1)+1:(i*(n+1)));
end

%% variables modification

Ta = xi(3);
Td0 = Td_in(1);
if (abs(u0(1))+abs(u0(2))) > (1*Thresh)
    y_Err = (x0(2)-xi(2));
    x_Err = (x0(1)-xi(1));
    XS = (y_Err/x_Err);
    Td0 = atan(XS); 
    if abs(Td0)>1.5
        Td0 = abs(Td0);
    end
end

% Td = zeros(N+1,1);
% Td(1) = Td0;
Td = Td0;
Diff_Real = zeros(n,N);
Dxi = zeros(2,N);
for i=1:N
    Diff_Real(1,i) = (xp(1,Agent_Num) - xp(1,i))*cos(Ta) + (xp(2,Agent_Num) - xp(2,i))*sin(Ta);
%     Tdi = Td_in(i+1);
%     Dxi(1,i) = xp(4,i)*cos(xp(3,i));
%     Dxi(2,i) = xp(4,i)*sin(xp(3,i));
%     if (abs(Dxi(1,i))+abs(Dxi(2,i))) > Thresh
%         y_Erri = xp(2,Agent_Num) - xp(2,i);
%         x_Erri = xp(1,Agent_Num) - xp(1,i);
%         Tdi = atan(y_Erri/x_Erri);
%         if abs(Tdi)>1.5
%             Tdi = abs(Tdi);
%         end
%     end
%     Diff_Real(2,i) = Ta - Tdi;
    Diff_Real(2,i) = Ta - xp(3,i);
    Diff_Real(3:4,i) = xp(4:5,Agent_Num) - xp(4:5,i); 
%     Td(i+1) = Tdi;
end
Diff_Real0 = zeros(n,1);
Diff_Real0(1) = (xp(1,Agent_Num) - x0(1))*cos(Ta) + (xp(2,Agent_Num) - x0(2))*sin(Ta);
Diff_Real0(2) = Ta - Td0; 
Diff_Real0(3:4) = xp(4:5,Agent_Num) - ui(1:n0);

Posi = xi(1)*cos(Ta) + xi(2)*sin(Ta);
Posd = x0(1)*cos(Ta) + x0(2)*sin(Ta);
xmi = [Posi;Ta;xi(4);xi(5)];
xm0 = [Posd;Td0]; 

%%

ep = zeros(n,1);
ep(1:2,1) = ep(1:2,1) + ( BN(Agent_Num,Agent_Num)*(-Diff_Real0(1:2)+Diff_Star_to0(1:2)) );
ep(3:4,1) = ep(3:4,1) + ( 1*(-Diff_Real0(3:4)+Diff_Star_to0(3:4)) );
for i=1:N            
    ep(1:n,1) = ep(1:n,1) + AN(Agent_Num,i)*(-Diff_Real(:,i)+Diff_Star_to_Other(:,i));
end

end

== matlab function CAMFC2_01_WMR01/Agent #3/Decenteralized Cooperaive Controller #3/Observer T#3 ==
  data: T_struct parameter; T input; DT_i output; epsilon input; epsilon_struct parameter; H parameter; BN parameter; AN parameter; T_i input; chi parameter; Upsilon_M parameter; epsilon_i output; N parameter; n parameter; Agent_Num input; Observer_Gain1 parameter
function [DT_i,epsilon_i] = fcn(T_struct,T,epsilon,epsilon_struct,H,BN,AN,T_i,chi,Upsilon_M,N,n,Agent_Num,Observer_Gain1)

T_struct(1).data = T.t1;
T_struct(2).data = T.t2;
T_struct(3).data = T.t3;
T_struct(4).data = T.t4;

epsilon_struct(1).data = epsilon.eps1;
epsilon_struct(2).data = epsilon.eps2;
epsilon_struct(3).data = epsilon.eps3;
epsilon_struct(4).data = epsilon.eps4;

epsilon_i = + BN(Agent_Num,Agent_Num)*(T_i - chi);
Sum2 = zeros(N+1,n);
for i=1:N
    epsilon_i = epsilon_i + ( AN(Agent_Num,i) * (T_i - T_struct(i).data) );  
    Sum2 = Sum2 + ( H(i,Agent_Num) * epsilon_struct(i).data );
end

Sum21 = abs(Sum2) + 0.1;
SGN2 = Sum2./Sum21;

DT_i = -Observer_Gain1*epsilon_i - SGN2*diag(Upsilon_M);

end

== matlab function CAMFC2_01_WMR01/Agent #3/Decenteralized Cooperaive Controller #3/Observer q#3 ==
  data: q input; Dq_i output; tau input; H parameter; BN parameter; AN parameter; q_i input; u0 input; U_dot0_M parameter; tau_i output; N parameter; Agent_Num input; Observer_Gain parameter; n parameter
function [Dq_i,tau_i] = fcn(q,tau,H,BN,AN,q_i,u0,U_dot0_M,N,Agent_Num,Observer_Gain,n)

tau_i = + BN(Agent_Num,Agent_Num)*(q_i - u0);
Sum2 = zeros(n,1);
for i=1:N
    tau_i = tau_i + ( AN(Agent_Num,i) * (q_i - q(((i-1)*n+1):n*i)) );  
    Sum2 = Sum2 + ( H(i,Agent_Num) * tau(((i-1)*n+1):n*i) );
end

Sum21 = abs(Sum2) + 0.01;
SGN2 = Sum2./Sum21;

Dq_i = -Observer_Gain*tau_i - diag(SGN2)*U_dot0_M;

end

== matlab function CAMFC2_01_WMR01/Agent #4/Decenteralized Cooperaive Controller #4/Main Controller #4 ==
  data: n parameter; n0 parameter; U output; R parameter; Q parameter; P_i input; e_i input; K parameter; Zeta_i input; BN parameter; A_hat_i input; u0 input; z0 input; DT_i input; T_i input; N parameter; H parameter; B parameter; g_hat input; Approx_U input; Agent_Num input; B_pseudo_inverse parameter; ui input; x input
function U = fcn(n,n0,R,Q,P_i,e_i,K,Zeta_i,BN,A_hat_i,u0,z0,DT_i,T_i,N,H,B,g_hat,Approx_U,Agent_Num,B_pseudo_inverse,ui,x)

D_eta_0 = DT_i(1,:)';

%%
z0_i = [z0;ui(1:n0)];
u0_i = u0;

%%
U2 = 1/2 * R * P_i * e_i; %Consensus Error
U6 = - BN(Agent_Num,Agent_Num)*(D_eta_0 - u0_i); %Connection to the leader
U7 = K * Zeta_i; %Consensus time-integral

U1 = zeros(n,1);
U3 = BN(Agent_Num,Agent_Num)*z0_i - e_i;
U4 = zeros(n,1);
U5 = zeros(n,1);
for i=1:N      
    if i~= Agent_Num
        U1 = U1 - (H(Agent_Num,i)*B*Approx_U((i-1)*n+1:(i*n),1)); %Observer on leader
    end
    U3 = U3 + (H(Agent_Num,i)*(2*x((i-1)*n+1:(i*n),1)) - T_i(i+1,:)'); %Formation parameters  
    U4 = U4 - (H(Agent_Num,i)*g_hat((i-1)*n+1:(i*n),1)); %nonlinear compensation 
    U5 = U5 + (H(Agent_Num,i)*DT_i(i+1,:)'); %Derivative of Formation parameters  
end
U3 = -A_hat_i * U3;
U8 = (2*Q - 3/4*R*P_i)*e_i;

U_input = U1 + U2 + U3 + U4 + U5 + U6 + U7 + U8;

U = B_pseudo_inverse * U_input / H(Agent_Num,Agent_Num);

end

== matlab function CAMFC2_01_WMR01/Agent #4/Decenteralized Cooperaive Controller #4/Module to compute Consensus Error #4 ==
  data: T_i input; xi input; x input; x0 input; ep output; AN parameter; BN parameter; N parameter; n parameter; n0 parameter; Agent_Num input; ui input; u0 input; Thresh parameter; xmi output; xm0 output; Td_in input; Td output
function [ep,xmi,xm0,Td] = fcn(T_i,xi,x,x0,AN,BN,N,n,n0,Agent_Num,ui,u0,Thresh,Td_in)

Diff_Star_to0 = (T_i((Agent_Num+1),:))';
Diff_Star_to_Other = (eye(n) * Diff_Star_to0 * ones(1,N))' - T_i(2:N+1,:);
Diff_Star_to_Other = Diff_Star_to_Other';

xp = zeros(n+1,N);
for i=1:N
    xp(1:n+1,i) = x((i-1)*(n+1)+1:(i*(n+1)));
end

%% variables modification

Ta = xi(3);
Td0 = Td_in(1);
if (abs(u0(1))+abs(u0(2))) > (1*Thresh)
    y_Err = (x0(2)-xi(2));
    x_Err = (x0(1)-xi(1));
    XS = (y_Err/x_Err);
    Td0 = atan(XS); 
    if abs(Td0)>1.5
        Td0 = abs(Td0);
    end
end

% Td = zeros(N+1,1);
% Td(1) = Td0;
Td = Td0;
Diff_Real = zeros(n,N);
Dxi = zeros(2,N);
for i=1:N
    Diff_Real(1,i) = (xp(1,Agent_Num) - xp(1,i))*cos(Ta) + (xp(2,Agent_Num) - xp(2,i))*sin(Ta);
%     Tdi = Td_in(i+1);
%     Dxi(1,i) = xp(4,i)*cos(xp(3,i));
%     Dxi(2,i) = xp(4,i)*sin(xp(3,i));
%     if (abs(Dxi(1,i))+abs(Dxi(2,i))) > Thresh
%         y_Erri = xp(2,Agent_Num) - xp(2,i);
%         x_Erri = xp(1,Agent_Num) - xp(1,i);
%         Tdi = atan(y_Erri/x_Erri);
%         if abs(Tdi)>1.5
%             Tdi = abs(Tdi);
%         end
%     end
%     Diff_Real(2,i) = Ta - Tdi;
    Diff_Real(2,i) = Ta - xp(3,i);
    Diff_Real(3:4,i) = xp(4:5,Agent_Num) - xp(4:5,i); 
%     Td(i+1) = Tdi;
end
Diff_Real0 = zeros(n,1);
Diff_Real0(1) = (xp(1,Agent_Num) - x0(1))*cos(Ta) + (xp(2,Agent_Num) - x0(2))*sin(Ta);
Diff_Real0(2) = Ta - Td0; 
Diff_Real0(3:4) = xp(4:5,Agent_Num) - ui(1:n0);

Posi = xi(1)*cos(Ta) + xi(2)*sin(Ta);
Posd = x0(1)*cos(Ta) + x0(2)*sin(Ta);
xmi = [Posi;Ta;xi(4);xi(5)];
xm0 = [Posd;Td0]; 

%%

ep = zeros(n,1);
ep(1:2,1) = ep(1:2,1) + ( BN(Agent_Num,Agent_Num)*(-Diff_Real0(1:2)+Diff_Star_to0(1:2)) );
ep(3:4,1) = ep(3:4,1) + ( 1*(-Diff_Real0(3:4)+Diff_Star_to0(3:4)) );
for i=1:N            
    ep(1:n,1) = ep(1:n,1) + AN(Agent_Num,i)*(-Diff_Real(:,i)+Diff_Star_to_Other(:,i));
end

end

== matlab function CAMFC2_01_WMR01/Agent #4/Decenteralized Cooperaive Controller #4/Observer T#4 ==
  data: T_struct parameter; T input; DT_i output; epsilon input; epsilon_struct parameter; H parameter; BN parameter; AN parameter; T_i input; chi parameter; Upsilon_M parameter; epsilon_i output; N parameter; n parameter; Agent_Num input; Observer_Gain1 parameter
function [DT_i,epsilon_i] = fcn(T_struct,T,epsilon,epsilon_struct,H,BN,AN,T_i,chi,Upsilon_M,N,n,Agent_Num,Observer_Gain1)

T_struct(1).data = T.t1;
T_struct(2).data = T.t2;
T_struct(3).data = T.t3;
T_struct(4).data = T.t4;

epsilon_struct(1).data = epsilon.eps1;
epsilon_struct(2).data = epsilon.eps2;
epsilon_struct(3).data = epsilon.eps3;
epsilon_struct(4).data = epsilon.eps4;

epsilon_i = + BN(Agent_Num,Agent_Num)*(T_i - chi);
Sum2 = zeros(N+1,n);
for i=1:N
    epsilon_i = epsilon_i + ( AN(Agent_Num,i) * (T_i - T_struct(i).data) );  
    Sum2 = Sum2 + ( H(i,Agent_Num) * epsilon_struct(i).data );
end

Sum21 = abs(Sum2) + 0.1;
SGN2 = Sum2./Sum21;

DT_i = -Observer_Gain1*epsilon_i - SGN2*diag(Upsilon_M);

end

== matlab function CAMFC2_01_WMR01/Agent #4/Decenteralized Cooperaive Controller #4/Observer q#4 ==
  data: q input; Dq_i output; tau input; H parameter; BN parameter; AN parameter; q_i input; u0 input; U_dot0_M parameter; tau_i output; N parameter; Agent_Num input; Observer_Gain parameter; n parameter
function [Dq_i,tau_i] = fcn(q,tau,H,BN,AN,q_i,u0,U_dot0_M,N,Agent_Num,Observer_Gain,n)

tau_i = + BN(Agent_Num,Agent_Num)*(q_i - u0);
Sum2 = zeros(n,1);
for i=1:N
    tau_i = tau_i + ( AN(Agent_Num,i) * (q_i - q(((i-1)*n+1):n*i)) );  
    Sum2 = Sum2 + ( H(i,Agent_Num) * tau(((i-1)*n+1):n*i) );
end

Sum21 = abs(Sum2) + 0.01;
SGN2 = Sum2./Sum21;

Dq_i = -Observer_Gain*tau_i - diag(SGN2)*U_dot0_M;

end
